simulink model "TSR_Scenario_002_cs"  (R2014b)
settings: Solver=ode5  SolverMode=SingleTasking  StartTime=0.0  StopTime=inf  FixedStep=1/100  RelTol=1e-3
PreLoadFcn:
  | mbxruntime.callbacks.PreLoadFcn(bdroot);
  | check_NUTS_defined;
  | 
  | assignin('base',['model_closed_' bdroot],false);
  | 
  | addpath('../includes_TSR/includes_TSR');
  | 
  | switch version('-release')
  | case {'2010a', '2010b', '2011a'}
  | addpath('../includes_TSR/ML2010b');
  | otherwise
  | addpath('../includes_TSR/ML2011b');
  | end
PostLoadFcn:
  | mbxruntime.callbacks.PostLoadFcn(bdroot);
InitFcn:
  | mbxruntime.callbacks.InitFcn(bdroot);;
  | 
  | addpath('..\includes_TSR');
StartFcn:
  | mbxruntime.callbacks.StartFcn(bdroot);
StopFcn:
  | mbxruntime.callbacks.StopFcn(bdroot);
model workspace: external: MAT-File .\TSR_Scenario_002_cs_hws.mat (data not in the file)
undefined symbols (not defined in the file or in its folder): InitImageOutputDir, mbxruntime, OrientationPitch, OrientationRoll, PositionX, PositionY, PositionZ, tabledata, warningInitialVelocity, x0
undefined symbols (not defined in the file): SteeringColumn, SteeringWheel, TSR_Scenario_002_cs_003e47b1b59594b6, TSR_Scenario_002_cs_023e87a31011dc74, TSR_Scenario_002_cs_048cb8409c90d9c6, TSR_Scenario_002_cs_106a0284aafa53e6, TSR_Scenario_002_cs_195b368d22a7f172, TSR_Scenario_002_cs_1e339fa5d680f213, TSR_Scenario_002_cs_26196a9fb104f950, TSR_Scenario_002_cs_261a709f6f453598, TSR_Scenario_002_cs_2ac3337370d0049d, TSR_Scenario_002_cs_2dc51e6a68b01b00, TSR_Scenario_002_cs_3460ff54d38ab2e2, TSR_Scenario_002_cs_42ea7d6e56bd6005, TSR_Scenario_002_cs_4dd419d6d2b56fc2, TSR_Scenario_002_cs_5316a21de09dff2f, TSR_Scenario_002_cs_538caacf3455966d, TSR_Scenario_002_cs_5b2cfdbcfc80811f, TSR_Scenario_002_cs_5ce0eafbb7a2dce7, TSR_Scenario_002_cs_62cdbf45c6f8824a, TSR_Scenario_002_cs_6bebc368eedff0bc, TSR_Scenario_002_cs_6d26481da4ed7e29, TSR_Scenario_002_cs_70c7e369ce6550e0, TSR_Scenario_002_cs_7a63051a1f311451, TSR_Scenario_002_cs_7d7dc8405f613c6d, TSR_Scenario_002_cs_7f65e296173485e8, TSR_Scenario_002_cs_87183cf6ff7bb4b6, TSR_Scenario_002_cs_8921b0da7ab80865, TSR_Scenario_002_cs_9495ce3a76763d1f, TSR_Scenario_002_cs_a679806a2fdc8099, TSR_Scenario_002_cs_Actros_1860_1_Path_pathUniqueID, TSR_Scenario_002_cs_Actros_2541_1_Path_pathUniqueID, TSR_Scenario_002_cs_Actros_2541_3_Path_pathUniqueID, TSR_Scenario_002_cs_Actros_2541_4_Path_pathUniqueID, TSR_Scenario_002_cs_adf24c93a9de8a4e, TSR_Scenario_002_cs_Audi_A8_1_Dynamics_Simple_initialPitch, TSR_Scenario_002_cs_Audi_A8_1_Dynamics_Simple_initialRoll, TSR_Scenario_002_cs_Audi_A8_1_Dynamics_Simple_initialX, TSR_Scenario_002_cs_Audi_A8_1_Dynamics_Simple_initialY, TSR_Scenario_002_cs_Audi_A8_1_Dynamics_Simple_initialYaw, TSR_Scenario_002_cs_Audi_A8_1_Dynamics_Simple_initialZ, TSR_Scenario_002_cs_b136c6ccb55f77db, TSR_Scenario_002_cs_ba4f809714c282b7, TSR_Scenario_002_cs_BMW_X5_1_Path_pathUniqueID, TSR_Scenario_002_cs_BMW_X5_1_SpeedProfile_speedProfileUniqueID, TSR_Scenario_002_cs_BMW_X5_2_Path_pathUniqueID, TSR_Scenario_002_cs_BMW_X5_2_SpeedProfile_speedProfileUniqueID, TSR_Scenario_002_cs_Citroen_C3_1_Path_pathUniqueID, TSR_Scenario_002_cs_Citroen_C3_2_Path_pathUniqueID, TSR_Scenario_002_cs_d8f275339b7082cf, TSR_Scenario_002_cs_Daf_95_1_Path_pathUniqueID, TSR_Scenario_002_cs_Daf_95_1_SpeedProfile_speedProfileUniqueID, TSR_Scenario_002_cs_dc019741510ce2f2, TSR_Scenario_002_cs_fdbc8aabe460b27c, TSR_Scenario_002_cs_Fiat_Bravo_1_Path_pathUniqueID, TSR_Scenario_002_cs_Ford_Fiesta_1_Path_pathUniqueID, TSR_Scenario_002_cs_Honda_Pan_European_1_Path_pathUniqueID, TSR_Scenario_002_cs_Mazda_RX8_1_Path_pathUniqueID, TSR_Scenario_002_cs_Nissan_Cabstar_1_Path_pathUniqueID, TSR_Scenario_002_cs_Nissan_Cabstar_2_Path_pathUniqueID ... (+9)
libraries: simulink_extras x82, simulink x23, PreScanSimulinkLibrary x11
(part 25 of 39)

== system TSR_Scenario_002_cs/VISUMatrixSignLights_HighwayOverhang_18/Actuator ==
  VISUMatrixSignLights_HighwayOverhang_18 : Inport  Tag=inport/VisuMatrixSignLights  SampleTime=1/100  BusOutputAsStruct=on
  DemuxVisuLights : Demux  Outputs=8
  LimiterVisuLights : Saturate  UpperLimit=1  LowerLimit=0
  visu_MatrixSign_31_Light_1 : S-Function  FunctionName=sfun_MaterialColorSelector  Parameters=mbxruntime.parameters.convert(UniqueID), mbxruntime.parameters.convert(ColorsObjectQuery), mbxruntime.parameters.convert(Colors),tabledata, TimeStep  EnableBusSupport=off  mask(PreScan Sink Block: VisuMatrixSignLights){UniqueID=1093, ColorsObjectQuery=child:name=MatrixSign_31/child:name=HighwayOverhang_18.MatrixSign_31.OrangeLightUpperLeft, Colors=[32   25    5  255   64   48    5  255   64   54    5  255    0    0    0  255; 45   34    0  255   45   34    0  255   45   34    0  255  306  229    5  255], TimeStep=1/100}
      mask prompts: UniqueID "Parent Unique Identifier"; ColorsObjectQuery "Query for Color Object"; Colors "Matrix of colors"; TimeStep "Simulink time step"
      mask help:
      | The VisuMatrixSignLights block provides a way to switch the lights on the matrix sign board on or off
      |
      | For more information, please click Help.
      mask init:
      | [tabledata] = mbxruntime.parameters.table(UniqueID,ColorsObjectQuery,Colors);
      mask Help: eval('openHelp(732)')
      mask Display: image(imread('RearLight.png'))
  visu_MatrixSign_31_Light_2 : S-Function  FunctionName=sfun_MaterialColorSelector  Parameters=mbxruntime.parameters.convert(UniqueID), mbxruntime.parameters.convert(ColorsObjectQuery), mbxruntime.parameters.convert(Colors),tabledata, TimeStep  EnableBusSupport=off  mask(PreScan Sink Block: VisuMatrixSignLights){UniqueID=1093, ColorsObjectQuery=child:name=MatrixSign_31/child:name=HighwayOverhang_18.MatrixSign_31.OrangeLightUpperRight, Colors=[32   25    5  255   64   48    5  255   64   54    5  255    0    0    0  255; 45   34    0  255   45   34    0  255   45   34    0  255  306  229    5  255], TimeStep=1/100}
      mask prompts: UniqueID "Parent Unique Identifier"; ColorsObjectQuery "Query for Color Object"; Colors "Matrix of colors"; TimeStep "Simulink time step"
      mask help:
      | The VisuMatrixSignLights block provides a way to switch the lights on the matrix sign board on or off
      |
      | For more information, please click Help.
      mask init:
      | [tabledata] = mbxruntime.parameters.table(UniqueID,ColorsObjectQuery,Colors);
      mask Help: eval('openHelp(732)')
      mask Display: image(imread('RearLight.png'))
  visu_MatrixSign_31_Light_3 : S-Function  FunctionName=sfun_MaterialColorSelector  Parameters=mbxruntime.parameters.convert(UniqueID), mbxruntime.parameters.convert(ColorsObjectQuery), mbxruntime.parameters.convert(Colors),tabledata, TimeStep  EnableBusSupport=off  mask(PreScan Sink Block: VisuMatrixSignLights){UniqueID=1093, ColorsObjectQuery=child:name=MatrixSign_31/child:name=HighwayOverhang_18.MatrixSign_31.OrangeLightLowerLeft, Colors=[32   25    5  255   64   48    5  255   64   54    5  255    0    0    0  255; 45   34    0  255   45   34    0  255   45   34    0  255  306  229    5  255], TimeStep=1/100}
      mask prompts: UniqueID "Parent Unique Identifier"; ColorsObjectQuery "Query for Color Object"; Colors "Matrix of colors"; TimeStep "Simulink time step"
      mask help:
      | The VisuMatrixSignLights block provides a way to switch the lights on the matrix sign board on or off
      |
      | For more information, please click Help.
      mask init:
      | [tabledata] = mbxruntime.parameters.table(UniqueID,ColorsObjectQuery,Colors);
      mask Help: eval('openHelp(732)')
      mask Display: image(imread('RearLight.png'))
  visu_MatrixSign_31_Light_4 : S-Function  FunctionName=sfun_MaterialColorSelector  Parameters=mbxruntime.parameters.convert(UniqueID), mbxruntime.parameters.convert(ColorsObjectQuery), mbxruntime.parameters.convert(Colors),tabledata, TimeStep  EnableBusSupport=off  mask(PreScan Sink Block: VisuMatrixSignLights){UniqueID=1093, ColorsObjectQuery=child:name=MatrixSign_31/child:name=HighwayOverhang_18.MatrixSign_31.OrangeLightLowerRight, Colors=[32   25    5  255   64   48    5  255   64   54    5  255    0    0    0  255; 45   34    0  255   45   34    0  255   45   34    0  255  306  229    5  255], TimeStep=1/100}
      mask prompts: UniqueID "Parent Unique Identifier"; ColorsObjectQuery "Query for Color Object"; Colors "Matrix of colors"; TimeStep "Simulink time step"
      mask help:
      | The VisuMatrixSignLights block provides a way to switch the lights on the matrix sign board on or off
      |
      | For more information, please click Help.
      mask init:
      | [tabledata] = mbxruntime.parameters.table(UniqueID,ColorsObjectQuery,Colors);
      mask Help: eval('openHelp(732)')
      mask Display: image(imread('RearLight.png'))
  visu_MatrixSign_32_Light_1 : S-Function  FunctionName=sfun_MaterialColorSelector  Parameters=mbxruntime.parameters.convert(UniqueID), mbxruntime.parameters.convert(ColorsObjectQuery), mbxruntime.parameters.convert(Colors),tabledata, TimeStep  EnableBusSupport=off  mask(PreScan Sink Block: VisuMatrixSignLights){UniqueID=1093, ColorsObjectQuery=child:name=MatrixSign_32/child:name=HighwayOverhang_18.MatrixSign_32.OrangeLightUpperLeft, Colors=[32   25    5  255   64   48    5  255   64   54    5  255    0    0    0  255; 45   34    0  255   45   34    0  255   45   34    0  255  306  229    5  255], TimeStep=1/100}
      mask prompts: UniqueID "Parent Unique Identifier"; ColorsObjectQuery "Query for Color Object"; Colors "Matrix of colors"; TimeStep "Simulink time step"
      mask help:
      | The VisuMatrixSignLights block provides a way to switch the lights on the matrix sign board on or off
      |
      | For more information, please click Help.
      mask init:
      | [tabledata] = mbxruntime.parameters.table(UniqueID,ColorsObjectQuery,Colors);
      mask Help: eval('openHelp(732)')
      mask Display: image(imread('RearLight.png'))
  visu_MatrixSign_32_Light_2 : S-Function  FunctionName=sfun_MaterialColorSelector  Parameters=mbxruntime.parameters.convert(UniqueID), mbxruntime.parameters.convert(ColorsObjectQuery), mbxruntime.parameters.convert(Colors),tabledata, TimeStep  EnableBusSupport=off  mask(PreScan Sink Block: VisuMatrixSignLights){UniqueID=1093, ColorsObjectQuery=child:name=MatrixSign_32/child:name=HighwayOverhang_18.MatrixSign_32.OrangeLightUpperRight, Colors=[32   25    5  255   64   48    5  255   64   54    5  255    0    0    0  255; 45   34    0  255   45   34    0  255   45   34    0  255  306  229    5  255], TimeStep=1/100}
      mask prompts: UniqueID "Parent Unique Identifier"; ColorsObjectQuery "Query for Color Object"; Colors "Matrix of colors"; TimeStep "Simulink time step"
      mask help:
      | The VisuMatrixSignLights block provides a way to switch the lights on the matrix sign board on or off
      |
      | For more information, please click Help.
      mask init:
      | [tabledata] = mbxruntime.parameters.table(UniqueID,ColorsObjectQuery,Colors);
      mask Help: eval('openHelp(732)')
      mask Display: image(imread('RearLight.png'))
  visu_MatrixSign_32_Light_3 : S-Function  FunctionName=sfun_MaterialColorSelector  Parameters=mbxruntime.parameters.convert(UniqueID), mbxruntime.parameters.convert(ColorsObjectQuery), mbxruntime.parameters.convert(Colors),tabledata, TimeStep  EnableBusSupport=off  mask(PreScan Sink Block: VisuMatrixSignLights){UniqueID=1093, ColorsObjectQuery=child:name=MatrixSign_32/child:name=HighwayOverhang_18.MatrixSign_32.OrangeLightLowerLeft, Colors=[32   25    5  255   64   48    5  255   64   54    5  255    0    0    0  255; 45   34    0  255   45   34    0  255   45   34    0  255  306  229    5  255], TimeStep=1/100}
      mask prompts: UniqueID "Parent Unique Identifier"; ColorsObjectQuery "Query for Color Object"; Colors "Matrix of colors"; TimeStep "Simulink time step"
      mask help:
      | The VisuMatrixSignLights block provides a way to switch the lights on the matrix sign board on or off
      |
      | For more information, please click Help.
      mask init:
      | [tabledata] = mbxruntime.parameters.table(UniqueID,ColorsObjectQuery,Colors);
      mask Help: eval('openHelp(732)')
      mask Display: image(imread('RearLight.png'))
  visu_MatrixSign_32_Light_4 : S-Function  FunctionName=sfun_MaterialColorSelector  Parameters=mbxruntime.parameters.convert(UniqueID), mbxruntime.parameters.convert(ColorsObjectQuery), mbxruntime.parameters.convert(Colors),tabledata, TimeStep  EnableBusSupport=off  mask(PreScan Sink Block: VisuMatrixSignLights){UniqueID=1093, ColorsObjectQuery=child:name=MatrixSign_32/child:name=HighwayOverhang_18.MatrixSign_32.OrangeLightLowerRight, Colors=[32   25    5  255   64   48    5  255   64   54    5  255    0    0    0  255; 45   34    0  255   45   34    0  255   45   34    0  255  306  229    5  255], TimeStep=1/100}
      mask prompts: UniqueID "Parent Unique Identifier"; ColorsObjectQuery "Query for Color Object"; Colors "Matrix of colors"; TimeStep "Simulink time step"
      mask help:
      | The VisuMatrixSignLights block provides a way to switch the lights on the matrix sign board on or off
      |
      | For more information, please click Help.
      mask init:
      | [tabledata] = mbxruntime.parameters.table(UniqueID,ColorsObjectQuery,Colors);
      mask Help: eval('openHelp(732)')
      mask Display: image(imread('RearLight.png'))
  wires:
  VISUMatrixSignLights_HighwayOverhang_18/1 -> LimiterVisuLights/1
  LimiterVisuLights/1 -> DemuxVisuLights/1
  DemuxVisuLights/1 -> visu_MatrixSign_31_Light_1/1
  DemuxVisuLights/2 -> visu_MatrixSign_31_Light_2/1
  DemuxVisuLights/3 -> visu_MatrixSign_31_Light_3/1
  DemuxVisuLights/4 -> visu_MatrixSign_31_Light_4/1
  DemuxVisuLights/5 -> visu_MatrixSign_32_Light_1/1
  DemuxVisuLights/6 -> visu_MatrixSign_32_Light_2/1
  DemuxVisuLights/7 -> visu_MatrixSign_32_Light_3/1
  DemuxVisuLights/8 -> visu_MatrixSign_32_Light_4/1

== system TSR_Scenario_002_cs/VISUMatrixSignLights_HighwayOverhang_19/Actuator ==
  VISUMatrixSignLights_HighwayOverhang_19 : Inport  Tag=inport/VisuMatrixSignLights  SampleTime=1/100  BusOutputAsStruct=on
  DemuxVisuLights : Demux  Outputs=8
  LimiterVisuLights : Saturate  UpperLimit=1  LowerLimit=0
  visu_MatrixSign_52_Light_1 : S-Function  FunctionName=sfun_MaterialColorSelector  Parameters=mbxruntime.parameters.convert(UniqueID), mbxruntime.parameters.convert(ColorsObjectQuery), mbxruntime.parameters.convert(Colors),tabledata, TimeStep  EnableBusSupport=off  mask(PreScan Sink Block: VisuMatrixSignLights){UniqueID=1095, ColorsObjectQuery=child:name=MatrixSign_52/child:name=HighwayOverhang_19.MatrixSign_52.OrangeLightUpperLeft, Colors=[32   25    5  255   64   48    5  255   64   54    5  255    0    0    0  255; 45   34    0  255   45   34    0  255   45   34    0  255  306  229    5  255], TimeStep=1/100}
      mask prompts: UniqueID "Parent Unique Identifier"; ColorsObjectQuery "Query for Color Object"; Colors "Matrix of colors"; TimeStep "Simulink time step"
      mask help:
      | The VisuMatrixSignLights block provides a way to switch the lights on the matrix sign board on or off
      |
      | For more information, please click Help.
      mask init:
      | [tabledata] = mbxruntime.parameters.table(UniqueID,ColorsObjectQuery,Colors);
      mask Help: eval('openHelp(732)')
      mask Display: image(imread('RearLight.png'))
  visu_MatrixSign_52_Light_2 : S-Function  FunctionName=sfun_MaterialColorSelector  Parameters=mbxruntime.parameters.convert(UniqueID), mbxruntime.parameters.convert(ColorsObjectQuery), mbxruntime.parameters.convert(Colors),tabledata, TimeStep  EnableBusSupport=off  mask(PreScan Sink Block: VisuMatrixSignLights){UniqueID=1095, ColorsObjectQuery=child:name=MatrixSign_52/child:name=HighwayOverhang_19.MatrixSign_52.OrangeLightUpperRight, Colors=[32   25    5  255   64   48    5  255   64   54    5  255    0    0    0  255; 45   34    0  255   45   34    0  255   45   34    0  255  306  229    5  255], TimeStep=1/100}
      mask prompts: UniqueID "Parent Unique Identifier"; ColorsObjectQuery "Query for Color Object"; Colors "Matrix of colors"; TimeStep "Simulink time step"
      mask help:
      | The VisuMatrixSignLights block provides a way to switch the lights on the matrix sign board on or off
      |
      | For more information, please click Help.
      mask init:
      | [tabledata] = mbxruntime.parameters.table(UniqueID,ColorsObjectQuery,Colors);
      mask Help: eval('openHelp(732)')
      mask Display: image(imread('RearLight.png'))
  visu_MatrixSign_52_Light_3 : S-Function  FunctionName=sfun_MaterialColorSelector  Parameters=mbxruntime.parameters.convert(UniqueID), mbxruntime.parameters.convert(ColorsObjectQuery), mbxruntime.parameters.convert(Colors),tabledata, TimeStep  EnableBusSupport=off  mask(PreScan Sink Block: VisuMatrixSignLights){UniqueID=1095, ColorsObjectQuery=child:name=MatrixSign_52/child:name=HighwayOverhang_19.MatrixSign_52.OrangeLightLowerLeft, Colors=[32   25    5  255   64   48    5  255   64   54    5  255    0    0    0  255; 45   34    0  255   45   34    0  255   45   34    0  255  306  229    5  255], TimeStep=1/100}
      mask prompts: UniqueID "Parent Unique Identifier"; ColorsObjectQuery "Query for Color Object"; Colors "Matrix of colors"; TimeStep "Simulink time step"
      mask help:
      | The VisuMatrixSignLights block provides a way to switch the lights on the matrix sign board on or off
      |
      | For more information, please click Help.
      mask init:
      | [tabledata] = mbxruntime.parameters.table(UniqueID,ColorsObjectQuery,Colors);
      mask Help: eval('openHelp(732)')
      mask Display: image(imread('RearLight.png'))
  visu_MatrixSign_52_Light_4 : S-Function  FunctionName=sfun_MaterialColorSelector  Parameters=mbxruntime.parameters.convert(UniqueID), mbxruntime.parameters.convert(ColorsObjectQuery), mbxruntime.parameters.convert(Colors),tabledata, TimeStep  EnableBusSupport=off  mask(PreScan Sink Block: VisuMatrixSignLights){UniqueID=1095, ColorsObjectQuery=child:name=MatrixSign_52/child:name=HighwayOverhang_19.MatrixSign_52.OrangeLightLowerRight, Colors=[32   25    5  255   64   48    5  255   64   54    5  255    0    0    0  255; 45   34    0  255   45   34    0  255   45   34    0  255  306  229    5  255], TimeStep=1/100}
      mask prompts: UniqueID "Parent Unique Identifier"; ColorsObjectQuery "Query for Color Object"; Colors "Matrix of colors"; TimeStep "Simulink time step"
      mask help:
      | The VisuMatrixSignLights block provides a way to switch the lights on the matrix sign board on or off
      |
      | For more information, please click Help.
      mask init:
      | [tabledata] = mbxruntime.parameters.table(UniqueID,ColorsObjectQuery,Colors);
      mask Help: eval('openHelp(732)')
      mask Display: image(imread('RearLight.png'))
  visu_MatrixSign_9_Light_1 : S-Function  FunctionName=sfun_MaterialColorSelector  Parameters=mbxruntime.parameters.convert(UniqueID), mbxruntime.parameters.convert(ColorsObjectQuery), mbxruntime.parameters.convert(Colors),tabledata, TimeStep  EnableBusSupport=off  mask(PreScan Sink Block: VisuMatrixSignLights){UniqueID=1095, ColorsObjectQuery=child:name=MatrixSign_9/child:name=HighwayOverhang_19.MatrixSign_9.OrangeLightUpperLeft, Colors=[32   25    5  255   64   48    5  255   64   54    5  255    0    0    0  255; 45   34    0  255   45   34    0  255   45   34    0  255  306  229    5  255], TimeStep=1/100}
      mask prompts: UniqueID "Parent Unique Identifier"; ColorsObjectQuery "Query for Color Object"; Colors "Matrix of colors"; TimeStep "Simulink time step"
      mask help:
      | The VisuMatrixSignLights block provides a way to switch the lights on the matrix sign board on or off
      |
      | For more information, please click Help.
      mask init:
      | [tabledata] = mbxruntime.parameters.table(UniqueID,ColorsObjectQuery,Colors);
      mask Help: eval('openHelp(732)')
      mask Display: image(imread('RearLight.png'))
  visu_MatrixSign_9_Light_2 : S-Function  FunctionName=sfun_MaterialColorSelector  Parameters=mbxruntime.parameters.convert(UniqueID), mbxruntime.parameters.convert(ColorsObjectQuery), mbxruntime.parameters.convert(Colors),tabledata, TimeStep  EnableBusSupport=off  mask(PreScan Sink Block: VisuMatrixSignLights){UniqueID=1095, ColorsObjectQuery=child:name=MatrixSign_9/child:name=HighwayOverhang_19.MatrixSign_9.OrangeLightUpperRight, Colors=[32   25    5  255   64   48    5  255   64   54    5  255    0    0    0  255; 45   34    0  255   45   34    0  255   45   34    0  255  306  229    5  255], TimeStep=1/100}
      mask prompts: UniqueID "Parent Unique Identifier"; ColorsObjectQuery "Query for Color Object"; Colors "Matrix of colors"; TimeStep "Simulink time step"
      mask help:
      | The VisuMatrixSignLights block provides a way to switch the lights on the matrix sign board on or off
      |
      | For more information, please click Help.
      mask init:
      | [tabledata] = mbxruntime.parameters.table(UniqueID,ColorsObjectQuery,Colors);
      mask Help: eval('openHelp(732)')
      mask Display: image(imread('RearLight.png'))
  visu_MatrixSign_9_Light_3 : S-Function  FunctionName=sfun_MaterialColorSelector  Parameters=mbxruntime.parameters.convert(UniqueID), mbxruntime.parameters.convert(ColorsObjectQuery), mbxruntime.parameters.convert(Colors),tabledata, TimeStep  EnableBusSupport=off  mask(PreScan Sink Block: VisuMatrixSignLights){UniqueID=1095, ColorsObjectQuery=child:name=MatrixSign_9/child:name=HighwayOverhang_19.MatrixSign_9.OrangeLightLowerLeft, Colors=[32   25    5  255   64   48    5  255   64   54    5  255    0    0    0  255; 45   34    0  255   45   34    0  255   45   34    0  255  306  229    5  255], TimeStep=1/100}
      mask prompts: UniqueID "Parent Unique Identifier"; ColorsObjectQuery "Query for Color Object"; Colors "Matrix of colors"; TimeStep "Simulink time step"
      mask help:
      | The VisuMatrixSignLights block provides a way to switch the lights on the matrix sign board on or off
      |
      | For more information, please click Help.
      mask init:
      | [tabledata] = mbxruntime.parameters.table(UniqueID,ColorsObjectQuery,Colors);
      mask Help: eval('openHelp(732)')
      mask Display: image(imread('RearLight.png'))
  visu_MatrixSign_9_Light_4 : S-Function  FunctionName=sfun_MaterialColorSelector  Parameters=mbxruntime.parameters.convert(UniqueID), mbxruntime.parameters.convert(ColorsObjectQuery), mbxruntime.parameters.convert(Colors),tabledata, TimeStep  EnableBusSupport=off  mask(PreScan Sink Block: VisuMatrixSignLights){UniqueID=1095, ColorsObjectQuery=child:name=MatrixSign_9/child:name=HighwayOverhang_19.MatrixSign_9.OrangeLightLowerRight, Colors=[32   25    5  255   64   48    5  255   64   54    5  255    0    0    0  255; 45   34    0  255   45   34    0  255   45   34    0  255  306  229    5  255], TimeStep=1/100}
      mask prompts: UniqueID "Parent Unique Identifier"; ColorsObjectQuery "Query for Color Object"; Colors "Matrix of colors"; TimeStep "Simulink time step"
      mask help:
      | The VisuMatrixSignLights block provides a way to switch the lights on the matrix sign board on or off
      |
      | For more information, please click Help.
      mask init:
      | [tabledata] = mbxruntime.parameters.table(UniqueID,ColorsObjectQuery,Colors);
      mask Help: eval('openHelp(732)')
      mask Display: image(imread('RearLight.png'))
  wires:
  VISUMatrixSignLights_HighwayOverhang_19/1 -> LimiterVisuLights/1
  LimiterVisuLights/1 -> DemuxVisuLights/1
  DemuxVisuLights/1 -> visu_MatrixSign_9_Light_1/1
  DemuxVisuLights/2 -> visu_MatrixSign_9_Light_2/1
  DemuxVisuLights/3 -> visu_MatrixSign_9_Light_3/1
  DemuxVisuLights/4 -> visu_MatrixSign_9_Light_4/1
  DemuxVisuLights/5 -> visu_MatrixSign_52_Light_1/1
  DemuxVisuLights/6 -> visu_MatrixSign_52_Light_2/1
  DemuxVisuLights/7 -> visu_MatrixSign_52_Light_3/1
  DemuxVisuLights/8 -> visu_MatrixSign_52_Light_4/1

== system TSR_Scenario_002_cs/VISUMatrixSignLights_HighwayOverhang_2/Actuator ==
  VISUMatrixSignLights_HighwayOverhang_2 : Inport  Tag=inport/VisuMatrixSignLights  SampleTime=1/100  BusOutputAsStruct=on
  DemuxVisuLights : Demux  Outputs=8
  LimiterVisuLights : Saturate  UpperLimit=1  LowerLimit=0
  visu_MatrixSign_14_Light_1 : S-Function  FunctionName=sfun_MaterialColorSelector  Parameters=mbxruntime.parameters.convert(UniqueID), mbxruntime.parameters.convert(ColorsObjectQuery), mbxruntime.parameters.convert(Colors),tabledata, TimeStep  EnableBusSupport=off  mask(PreScan Sink Block: VisuMatrixSignLights){UniqueID=432, ColorsObjectQuery=child:name=MatrixSign_14/child:name=HighwayOverhang_2.MatrixSign_14.OrangeLightUpperLeft, Colors=[32   25    5  255   64   48    5  255   64   54    5  255    0    0    0  255; 45   34    0  255   45   34    0  255   45   34    0  255  306  229    5  255], TimeStep=1/100}
      mask prompts: UniqueID "Parent Unique Identifier"; ColorsObjectQuery "Query for Color Object"; Colors "Matrix of colors"; TimeStep "Simulink time step"
      mask help:
      | The VisuMatrixSignLights block provides a way to switch the lights on the matrix sign board on or off
      |
      | For more information, please click Help.
      mask init:
      | [tabledata] = mbxruntime.parameters.table(UniqueID,ColorsObjectQuery,Colors);
      mask Help: eval('openHelp(732)')
      mask Display: image(imread('RearLight.png'))
  visu_MatrixSign_14_Light_2 : S-Function  FunctionName=sfun_MaterialColorSelector  Parameters=mbxruntime.parameters.convert(UniqueID), mbxruntime.parameters.convert(ColorsObjectQuery), mbxruntime.parameters.convert(Colors),tabledata, TimeStep  EnableBusSupport=off  mask(PreScan Sink Block: VisuMatrixSignLights){UniqueID=432, ColorsObjectQuery=child:name=MatrixSign_14/child:name=HighwayOverhang_2.MatrixSign_14.OrangeLightUpperRight, Colors=[32   25    5  255   64   48    5  255   64   54    5  255    0    0    0  255; 45   34    0  255   45   34    0  255   45   34    0  255  306  229    5  255], TimeStep=1/100}
      mask prompts: UniqueID "Parent Unique Identifier"; ColorsObjectQuery "Query for Color Object"; Colors "Matrix of colors"; TimeStep "Simulink time step"
      mask help:
      | The VisuMatrixSignLights block provides a way to switch the lights on the matrix sign board on or off
      |
      | For more information, please click Help.
      mask init:
      | [tabledata] = mbxruntime.parameters.table(UniqueID,ColorsObjectQuery,Colors);
      mask Help: eval('openHelp(732)')
      mask Display: image(imread('RearLight.png'))
  visu_MatrixSign_14_Light_3 : S-Function  FunctionName=sfun_MaterialColorSelector  Parameters=mbxruntime.parameters.convert(UniqueID), mbxruntime.parameters.convert(ColorsObjectQuery), mbxruntime.parameters.convert(Colors),tabledata, TimeStep  EnableBusSupport=off  mask(PreScan Sink Block: VisuMatrixSignLights){UniqueID=432, ColorsObjectQuery=child:name=MatrixSign_14/child:name=HighwayOverhang_2.MatrixSign_14.OrangeLightLowerLeft, Colors=[32   25    5  255   64   48    5  255   64   54    5  255    0    0    0  255; 45   34    0  255   45   34    0  255   45   34    0  255  306  229    5  255], TimeStep=1/100}
      mask prompts: UniqueID "Parent Unique Identifier"; ColorsObjectQuery "Query for Color Object"; Colors "Matrix of colors"; TimeStep "Simulink time step"
      mask help:
      | The VisuMatrixSignLights block provides a way to switch the lights on the matrix sign board on or off
      |
      | For more information, please click Help.
      mask init:
      | [tabledata] = mbxruntime.parameters.table(UniqueID,ColorsObjectQuery,Colors);
      mask Help: eval('openHelp(732)')
      mask Display: image(imread('RearLight.png'))
  visu_MatrixSign_14_Light_4 : S-Function  FunctionName=sfun_MaterialColorSelector  Parameters=mbxruntime.parameters.convert(UniqueID), mbxruntime.parameters.convert(ColorsObjectQuery), mbxruntime.parameters.convert(Colors),tabledata, TimeStep  EnableBusSupport=off  mask(PreScan Sink Block: VisuMatrixSignLights){UniqueID=432, ColorsObjectQuery=child:name=MatrixSign_14/child:name=HighwayOverhang_2.MatrixSign_14.OrangeLightLowerRight, Colors=[32   25    5  255   64   48    5  255   64   54    5  255    0    0    0  255; 45   34    0  255   45   34    0  255   45   34    0  255  306  229    5  255], TimeStep=1/100}
      mask prompts: UniqueID "Parent Unique Identifier"; ColorsObjectQuery "Query for Color Object"; Colors "Matrix of colors"; TimeStep "Simulink time step"
      mask help:
      | The VisuMatrixSignLights block provides a way to switch the lights on the matrix sign board on or off
      |
      | For more information, please click Help.
      mask init:
      | [tabledata] = mbxruntime.parameters.table(UniqueID,ColorsObjectQuery,Colors);
      mask Help: eval('openHelp(732)')
      mask Display: image(imread('RearLight.png'))
  visu_MatrixSign_2_Light_1 : S-Function  FunctionName=sfun_MaterialColorSelector  Parameters=mbxruntime.parameters.convert(UniqueID), mbxruntime.parameters.convert(ColorsObjectQuery), mbxruntime.parameters.convert(Colors),tabledata, TimeStep  EnableBusSupport=off  mask(PreScan Sink Block: VisuMatrixSignLights){UniqueID=432, ColorsObjectQuery=child:name=MatrixSign_2/child:name=HighwayOverhang_2.MatrixSign_2.OrangeLightUpperLeft, Colors=[32   25    5  255   64   48    5  255   64   54    5  255    0    0    0  255; 45   34    0  255   45   34    0  255   45   34    0  255  306  229    5  255], TimeStep=1/100}
      mask prompts: UniqueID "Parent Unique Identifier"; ColorsObjectQuery "Query for Color Object"; Colors "Matrix of colors"; TimeStep "Simulink time step"
      mask help:
      | The VisuMatrixSignLights block provides a way to switch the lights on the matrix sign board on or off
      |
      | For more information, please click Help.
      mask init:
      | [tabledata] = mbxruntime.parameters.table(UniqueID,ColorsObjectQuery,Colors);
      mask Help: eval('openHelp(732)')
      mask Display: image(imread('RearLight.png'))
  visu_MatrixSign_2_Light_2 : S-Function  FunctionName=sfun_MaterialColorSelector  Parameters=mbxruntime.parameters.convert(UniqueID), mbxruntime.parameters.convert(ColorsObjectQuery), mbxruntime.parameters.convert(Colors),tabledata, TimeStep  EnableBusSupport=off  mask(PreScan Sink Block: VisuMatrixSignLights){UniqueID=432, ColorsObjectQuery=child:name=MatrixSign_2/child:name=HighwayOverhang_2.MatrixSign_2.OrangeLightUpperRight, Colors=[32   25    5  255   64   48    5  255   64   54    5  255    0    0    0  255; 45   34    0  255   45   34    0  255   45   34    0  255  306  229    5  255], TimeStep=1/100}
      mask prompts: UniqueID "Parent Unique Identifier"; ColorsObjectQuery "Query for Color Object"; Colors "Matrix of colors"; TimeStep "Simulink time step"
      mask help:
      | The VisuMatrixSignLights block provides a way to switch the lights on the matrix sign board on or off
      |
      | For more information, please click Help.
      mask init:
      | [tabledata] = mbxruntime.parameters.table(UniqueID,ColorsObjectQuery,Colors);
      mask Help: eval('openHelp(732)')
      mask Display: image(imread('RearLight.png'))
  visu_MatrixSign_2_Light_3 : S-Function  FunctionName=sfun_MaterialColorSelector  Parameters=mbxruntime.parameters.convert(UniqueID), mbxruntime.parameters.convert(ColorsObjectQuery), mbxruntime.parameters.convert(Colors),tabledata, TimeStep  EnableBusSupport=off  mask(PreScan Sink Block: VisuMatrixSignLights){UniqueID=432, ColorsObjectQuery=child:name=MatrixSign_2/child:name=HighwayOverhang_2.MatrixSign_2.OrangeLightLowerLeft, Colors=[32   25    5  255   64   48    5  255   64   54    5  255    0    0    0  255; 45   34    0  255   45   34    0  255   45   34    0  255  306  229    5  255], TimeStep=1/100}
      mask prompts: UniqueID "Parent Unique Identifier"; ColorsObjectQuery "Query for Color Object"; Colors "Matrix of colors"; TimeStep "Simulink time step"
      mask help:
      | The VisuMatrixSignLights block provides a way to switch the lights on the matrix sign board on or off
      |
      | For more information, please click Help.
      mask init:
      | [tabledata] = mbxruntime.parameters.table(UniqueID,ColorsObjectQuery,Colors);
      mask Help: eval('openHelp(732)')
      mask Display: image(imread('RearLight.png'))
  visu_MatrixSign_2_Light_4 : S-Function  FunctionName=sfun_MaterialColorSelector  Parameters=mbxruntime.parameters.convert(UniqueID), mbxruntime.parameters.convert(ColorsObjectQuery), mbxruntime.parameters.convert(Colors),tabledata, TimeStep  EnableBusSupport=off  mask(PreScan Sink Block: VisuMatrixSignLights){UniqueID=432, ColorsObjectQuery=child:name=MatrixSign_2/child:name=HighwayOverhang_2.MatrixSign_2.OrangeLightLowerRight, Colors=[32   25    5  255   64   48    5  255   64   54    5  255    0    0    0  255; 45   34    0  255   45   34    0  255   45   34    0  255  306  229    5  255], TimeStep=1/100}
      mask prompts: UniqueID "Parent Unique Identifier"; ColorsObjectQuery "Query for Color Object"; Colors "Matrix of colors"; TimeStep "Simulink time step"
      mask help:
      | The VisuMatrixSignLights block provides a way to switch the lights on the matrix sign board on or off
      |
      | For more information, please click Help.
      mask init:
      | [tabledata] = mbxruntime.parameters.table(UniqueID,ColorsObjectQuery,Colors);
      mask Help: eval('openHelp(732)')
      mask Display: image(imread('RearLight.png'))
  wires:
  VISUMatrixSignLights_HighwayOverhang_2/1 -> LimiterVisuLights/1
  LimiterVisuLights/1 -> DemuxVisuLights/1
  DemuxVisuLights/1 -> visu_MatrixSign_14_Light_1/1
  DemuxVisuLights/2 -> visu_MatrixSign_14_Light_2/1
  DemuxVisuLights/3 -> visu_MatrixSign_14_Light_3/1
  DemuxVisuLights/4 -> visu_MatrixSign_14_Light_4/1
  DemuxVisuLights/5 -> visu_MatrixSign_2_Light_1/1
  DemuxVisuLights/6 -> visu_MatrixSign_2_Light_2/1
  DemuxVisuLights/7 -> visu_MatrixSign_2_Light_3/1
  DemuxVisuLights/8 -> visu_MatrixSign_2_Light_4/1

== system TSR_Scenario_002_cs/VISUMatrixSignLights_HighwayOverhang_20/Actuator ==
  VISUMatrixSignLights_HighwayOverhang_20 : Inport  Tag=inport/VisuMatrixSignLights  SampleTime=1/100  BusOutputAsStruct=on
  DemuxVisuLights : Demux  Outputs=8
  LimiterVisuLights : Saturate  UpperLimit=1  LowerLimit=0
  visu_MatrixSign_33_Light_1 : S-Function  FunctionName=sfun_MaterialColorSelector  Parameters=mbxruntime.parameters.convert(UniqueID), mbxruntime.parameters.convert(ColorsObjectQuery), mbxruntime.parameters.convert(Colors),tabledata, TimeStep  EnableBusSupport=off  mask(PreScan Sink Block: VisuMatrixSignLights){UniqueID=1094, ColorsObjectQuery=child:name=MatrixSign_33/child:name=HighwayOverhang_20.MatrixSign_33.OrangeLightUpperLeft, Colors=[32   25    5  255   64   48    5  255   64   54    5  255    0    0    0  255; 45   34    0  255   45   34    0  255   45   34    0  255  306  229    5  255], TimeStep=1/100}
      mask prompts: UniqueID "Parent Unique Identifier"; ColorsObjectQuery "Query for Color Object"; Colors "Matrix of colors"; TimeStep "Simulink time step"
      mask help:
      | The VisuMatrixSignLights block provides a way to switch the lights on the matrix sign board on or off
      |
      | For more information, please click Help.
      mask init:
      | [tabledata] = mbxruntime.parameters.table(UniqueID,ColorsObjectQuery,Colors);
      mask Help: eval('openHelp(732)')
      mask Display: image(imread('RearLight.png'))
  visu_MatrixSign_33_Light_2 : S-Function  FunctionName=sfun_MaterialColorSelector  Parameters=mbxruntime.parameters.convert(UniqueID), mbxruntime.parameters.convert(ColorsObjectQuery), mbxruntime.parameters.convert(Colors),tabledata, TimeStep  EnableBusSupport=off  mask(PreScan Sink Block: VisuMatrixSignLights){UniqueID=1094, ColorsObjectQuery=child:name=MatrixSign_33/child:name=HighwayOverhang_20.MatrixSign_33.OrangeLightUpperRight, Colors=[32   25    5  255   64   48    5  255   64   54    5  255    0    0    0  255; 45   34    0  255   45   34    0  255   45   34    0  255  306  229    5  255], TimeStep=1/100}
      mask prompts: UniqueID "Parent Unique Identifier"; ColorsObjectQuery "Query for Color Object"; Colors "Matrix of colors"; TimeStep "Simulink time step"
      mask help:
      | The VisuMatrixSignLights block provides a way to switch the lights on the matrix sign board on or off
      |
      | For more information, please click Help.
      mask init:
      | [tabledata] = mbxruntime.parameters.table(UniqueID,ColorsObjectQuery,Colors);
      mask Help: eval('openHelp(732)')
      mask Display: image(imread('RearLight.png'))
  visu_MatrixSign_33_Light_3 : S-Function  FunctionName=sfun_MaterialColorSelector  Parameters=mbxruntime.parameters.convert(UniqueID), mbxruntime.parameters.convert(ColorsObjectQuery), mbxruntime.parameters.convert(Colors),tabledata, TimeStep  EnableBusSupport=off  mask(PreScan Sink Block: VisuMatrixSignLights){UniqueID=1094, ColorsObjectQuery=child:name=MatrixSign_33/child:name=HighwayOverhang_20.MatrixSign_33.OrangeLightLowerLeft, Colors=[32   25    5  255   64   48    5  255   64   54    5  255    0    0    0  255; 45   34    0  255   45   34    0  255   45   34    0  255  306  229    5  255], TimeStep=1/100}
      mask prompts: UniqueID "Parent Unique Identifier"; ColorsObjectQuery "Query for Color Object"; Colors "Matrix of colors"; TimeStep "Simulink time step"
      mask help:
      | The VisuMatrixSignLights block provides a way to switch the lights on the matrix sign board on or off
      |
      | For more information, please click Help.
      mask init:
      | [tabledata] = mbxruntime.parameters.table(UniqueID,ColorsObjectQuery,Colors);
      mask Help: eval('openHelp(732)')
      mask Display: image(imread('RearLight.png'))
  visu_MatrixSign_33_Light_4 : S-Function  FunctionName=sfun_MaterialColorSelector  Parameters=mbxruntime.parameters.convert(UniqueID), mbxruntime.parameters.convert(ColorsObjectQuery), mbxruntime.parameters.convert(Colors),tabledata, TimeStep  EnableBusSupport=off  mask(PreScan Sink Block: VisuMatrixSignLights){UniqueID=1094, ColorsObjectQuery=child:name=MatrixSign_33/child:name=HighwayOverhang_20.MatrixSign_33.OrangeLightLowerRight, Colors=[32   25    5  255   64   48    5  255   64   54    5  255    0    0    0  255; 45   34    0  255   45   34    0  255   45   34    0  255  306  229    5  255], TimeStep=1/100}
      mask prompts: UniqueID "Parent Unique Identifier"; ColorsObjectQuery "Query for Color Object"; Colors "Matrix of colors"; TimeStep "Simulink time step"
      mask help:
      | The VisuMatrixSignLights block provides a way to switch the lights on the matrix sign board on or off
      |
      | For more information, please click Help.
      mask init:
      | [tabledata] = mbxruntime.parameters.table(UniqueID,ColorsObjectQuery,Colors);
      mask Help: eval('openHelp(732)')
      mask Display: image(imread('RearLight.png'))
  visu_MatrixSign_34_Light_1 : S-Function  FunctionName=sfun_MaterialColorSelector  Parameters=mbxruntime.parameters.convert(UniqueID), mbxruntime.parameters.convert(ColorsObjectQuery), mbxruntime.parameters.convert(Colors),tabledata, TimeStep  EnableBusSupport=off  mask(PreScan Sink Block: VisuMatrixSignLights){UniqueID=1094, ColorsObjectQuery=child:name=MatrixSign_34/child:name=HighwayOverhang_20.MatrixSign_34.OrangeLightUpperLeft, Colors=[32   25    5  255   64   48    5  255   64   54    5  255    0    0    0  255; 45   34    0  255   45   34    0  255   45   34    0  255  306  229    5  255], TimeStep=1/100}
      mask prompts: UniqueID "Parent Unique Identifier"; ColorsObjectQuery "Query for Color Object"; Colors "Matrix of colors"; TimeStep "Simulink time step"
      mask help:
      | The VisuMatrixSignLights block provides a way to switch the lights on the matrix sign board on or off
      |
      | For more information, please click Help.
      mask init:
      | [tabledata] = mbxruntime.parameters.table(UniqueID,ColorsObjectQuery,Colors);
      mask Help: eval('openHelp(732)')
      mask Display: image(imread('RearLight.png'))
  visu_MatrixSign_34_Light_2 : S-Function  FunctionName=sfun_MaterialColorSelector  Parameters=mbxruntime.parameters.convert(UniqueID), mbxruntime.parameters.convert(ColorsObjectQuery), mbxruntime.parameters.convert(Colors),tabledata, TimeStep  EnableBusSupport=off  mask(PreScan Sink Block: VisuMatrixSignLights){UniqueID=1094, ColorsObjectQuery=child:name=MatrixSign_34/child:name=HighwayOverhang_20.MatrixSign_34.OrangeLightUpperRight, Colors=[32   25    5  255   64   48    5  255   64   54    5  255    0    0    0  255; 45   34    0  255   45   34    0  255   45   34    0  255  306  229    5  255], TimeStep=1/100}
      mask prompts: UniqueID "Parent Unique Identifier"; ColorsObjectQuery "Query for Color Object"; Colors "Matrix of colors"; TimeStep "Simulink time step"
      mask help:
      | The VisuMatrixSignLights block provides a way to switch the lights on the matrix sign board on or off
      |
      | For more information, please click Help.
      mask init:
      | [tabledata] = mbxruntime.parameters.table(UniqueID,ColorsObjectQuery,Colors);
      mask Help: eval('openHelp(732)')
      mask Display: image(imread('RearLight.png'))
  visu_MatrixSign_34_Light_3 : S-Function  FunctionName=sfun_MaterialColorSelector  Parameters=mbxruntime.parameters.convert(UniqueID), mbxruntime.parameters.convert(ColorsObjectQuery), mbxruntime.parameters.convert(Colors),tabledata, TimeStep  EnableBusSupport=off  mask(PreScan Sink Block: VisuMatrixSignLights){UniqueID=1094, ColorsObjectQuery=child:name=MatrixSign_34/child:name=HighwayOverhang_20.MatrixSign_34.OrangeLightLowerLeft, Colors=[32   25    5  255   64   48    5  255   64   54    5  255    0    0    0  255; 45   34    0  255   45   34    0  255   45   34    0  255  306  229    5  255], TimeStep=1/100}
      mask prompts: UniqueID "Parent Unique Identifier"; ColorsObjectQuery "Query for Color Object"; Colors "Matrix of colors"; TimeStep "Simulink time step"
      mask help:
      | The VisuMatrixSignLights block provides a way to switch the lights on the matrix sign board on or off
      |
      | For more information, please click Help.
      mask init:
      | [tabledata] = mbxruntime.parameters.table(UniqueID,ColorsObjectQuery,Colors);
      mask Help: eval('openHelp(732)')
      mask Display: image(imread('RearLight.png'))
  visu_MatrixSign_34_Light_4 : S-Function  FunctionName=sfun_MaterialColorSelector  Parameters=mbxruntime.parameters.convert(UniqueID), mbxruntime.parameters.convert(ColorsObjectQuery), mbxruntime.parameters.convert(Colors),tabledata, TimeStep  EnableBusSupport=off  mask(PreScan Sink Block: VisuMatrixSignLights){UniqueID=1094, ColorsObjectQuery=child:name=MatrixSign_34/child:name=HighwayOverhang_20.MatrixSign_34.OrangeLightLowerRight, Colors=[32   25    5  255   64   48    5  255   64   54    5  255    0    0    0  255; 45   34    0  255   45   34    0  255   45   34    0  255  306  229    5  255], TimeStep=1/100}
      mask prompts: UniqueID "Parent Unique Identifier"; ColorsObjectQuery "Query for Color Object"; Colors "Matrix of colors"; TimeStep "Simulink time step"
      mask help:
      | The VisuMatrixSignLights block provides a way to switch the lights on the matrix sign board on or off
      |
      | For more information, please click Help.
      mask init:
      | [tabledata] = mbxruntime.parameters.table(UniqueID,ColorsObjectQuery,Colors);
      mask Help: eval('openHelp(732)')
      mask Display: image(imread('RearLight.png'))
  wires:
  VISUMatrixSignLights_HighwayOverhang_20/1 -> LimiterVisuLights/1
  LimiterVisuLights/1 -> DemuxVisuLights/1
  DemuxVisuLights/1 -> visu_MatrixSign_33_Light_1/1
  DemuxVisuLights/2 -> visu_MatrixSign_33_Light_2/1
  DemuxVisuLights/3 -> visu_MatrixSign_33_Light_3/1
  DemuxVisuLights/4 -> visu_MatrixSign_33_Light_4/1
  DemuxVisuLights/5 -> visu_MatrixSign_34_Light_1/1
  DemuxVisuLights/6 -> visu_MatrixSign_34_Light_2/1
  DemuxVisuLights/7 -> visu_MatrixSign_34_Light_3/1
  DemuxVisuLights/8 -> visu_MatrixSign_34_Light_4/1
